simulink model "servo_motors_simulink"  (R2024b)
settings: Solver=VariableStepAuto  StartTime=0.0  StopTime=100  RelTol=1e-3
values from neighbouring files (symbols this model uses):
  Beq = Bm + Bt + B*r^2    (= 1)    [servo_motors_matlab.m]
  Jeq = Jm + Jt + M*r^2    (= 1)    [servo_motors_matlab.m]
  Kt = 1    [servo_motors_matlab.m]
libraries: slpidlib x4
settings Model: Creator=mstfy  LastModifiedBy=mstfy

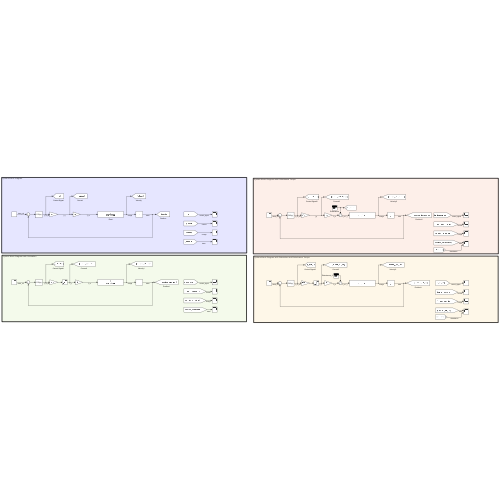
[thumbnail: Simulink's stored preview of the top-level diagram]
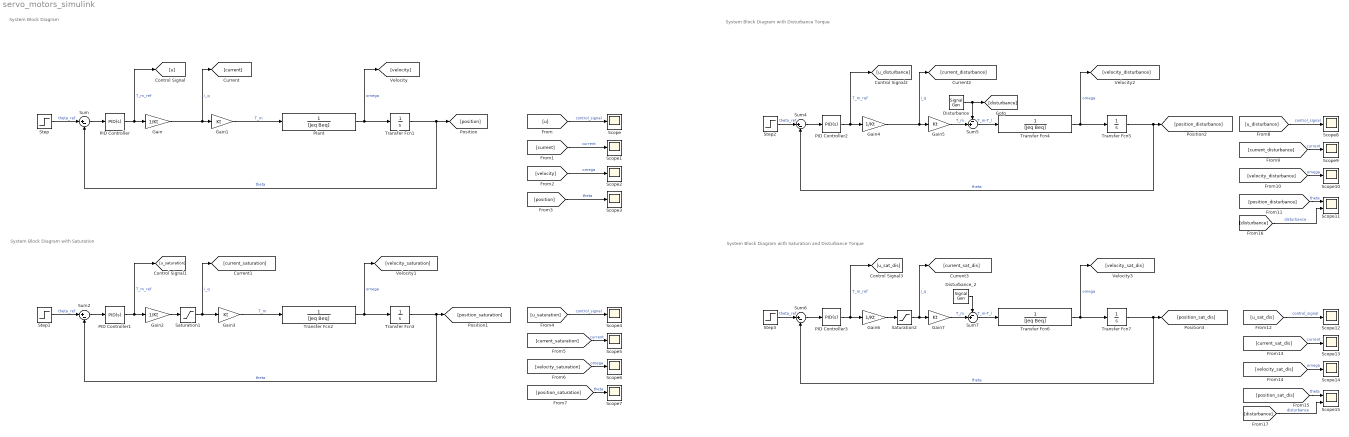
== system servo_motors_simulink ==
  note: System Block Diagram with Saturation
  note: System Block Diagram
  note: System Block Diagram with Disturbance Torque
  note: System Block Diagram with Saturation and Disturbance Torque
  Disturbance : SignalGenerator  WaveForm=square  Frequency=0.125  Units=rad/sec
  Disturbance_2 : SignalGenerator  WaveForm=square  Amplitude=0.5  Frequency=0.125  Units=rad/sec
  Gain{,2,4,6} (4 alike) : Gain  Gain=1/Kt
  Gain{1,3,5,7} (4 alike) : Gain  Gain=Kt
  PID Controller{,1..3} (4 alike) : slpidlib/PID Controller  Controller=PID  Form=Parallel  TimeDomain=Continuous-time  UseExternalTs=off  SampleTime=-1  IntegratorMethod=Forward Euler  FilterMethod=Forward Euler  ControllerParametersSource=internal  P=2.75  I=0.625  UseKiTs=off  D=2.5  UseExternalDerivativeSource=off  N=100  UseFilter=on  TunerSelectOption=Transfer Function Based (PID Tuner App)  InitialConditionSource=internal  InitialConditionForIntegrator=0  InitialConditionForFilter=0  DifferentiatorICPrevScaledInput=0  ExternalReset=none  TrackingMode=off  Kt=1  LimitOutput=off  SatLimitsSource=internal  UpperSaturationLimit=inf  LowerSaturationLimit=-inf  LinearizeAsGain=on  AntiWindupMode=none  Kb=1  LimitIntegrator=off  UpperIntegratorSaturationLimit=inf  LowerIntegratorSaturationLimit=-inf  POutMin=[]  POutMax=[]  IOutMin=[]  IOutMax=[]  DOutMin=[]  DOutMax=[]  NOutMin=[]  NOutMax=[]  SumOutMin=[]  SumOutMax=[]  SaturationOutMin=[]  SaturationOutMax=[]  PParamMin=[]  PParamMax=[]  IParamMin=[]  IParamMax=[]  DParamMin=[]  DParamMax=[]  NParamMin=[]  NParamMax=[]  KbParamMin=[]  KbParamMax=[]  KtParamMin=[]  KtParamMax=[]  KbOutMin=[]  KbOutMax=[]  KtOutMin=[]  KtOutMax=[]  IntegratorOutMin=[]  IntegratorOutMax=[]  FilterOutMin=[]  FilterOutMax=[]  SumI1OutMin=[]  SumI1OutMax=[]  SumI2OutMin=[]  SumI2OutMax=[]  SumI3OutMin=[]  SumI3OutMax=[]  SumI4OutMin=[]  SumI4OutMax=[]  SumDOutMin=[]  SumDOutMax=[]  DifferentiatorOutMin=[]  DifferentiatorOutMax=[]  FilterDiffOutCoefMin=[]  FilterDiffOutCoefMax=[]  ReciprocalOutMin=[]  ReciprocalOutMax=[]  SumDenOutMin=[]  SumDenOutMax=[]  SumNumOutMin=[]  SumNumOutMax=[]  DivideOutMin=[]  DivideOutMax=[]  UdiffTsProdOutMin=[]  UdiffTsProdOutMax=[]  NTsProdOutMin=[]  NTsProdOutMax=[]  UintegralTsProdOutMin=[]  UintegralTsProdOutMax=[]  UngainTsProdOutMin=[]  UngainTsProdOutMax=[]  ClampingZeroOutDataTypeStr=Inherit: Inherit via back propagation  ClampingZeroOutMin=[]  ClampingZeroOutMax=[]  FilterDenConstantOutDataTypeStr=Inherit: Inherit via back propagation  FilterDenConstantOutMin=[]  FilterDenConstantOutMax=[]  PCopyOutDataTypeStr=Inherit: Inherit via back propagation  PCopyOutMin=[]  PCopyOutMax=[]  NCopyOutDataTypeStr=Inherit: Inherit via back propagation  NCopyOutMin=[]  NCopyOutMax=[]  IntegratorContinuousStateAttributes=''  IntegratorStateMustResolveToSignalObject=off  IntegratorRTWStateStorageClass=Auto  FilterContinuousStateAttributes=''  FilterStateMustResolveToSignalObject=off  FilterRTWStateStorageClass=Auto  ParallelPVariant=InternalParameters  IdealPVariant=Disabled  IVariant=InternalParameters  DVariant=InternalParameters  IntegratorVariant=Continuous  SatVariant=Disabled  AWVariant=Passthrough  PCopyVariant=Disabled  TRVariant=Disabled  FdbkBlocksVariant=Forward  IdealPFdbkVariant=Disabled  SatFdbkVariant=Disabled  DerivativeFilterVariant=ContFilter  NVariant=InternalParameters  NCopyVariant=Disabled  FilterICVariant=InternalICsFilter  IntegratorICVariant=InternalICs  ExternalResetVariant=Disabled  TRSumVariant=Passthrough  SumFdbkVariant=Disabled  SumVariant=Sum_PID  TsampFilterVariant=InternalTs  TsampNgainVariant=Passthrough  TsampIntegralVariant=Disabled_SignalSpec  ExternalSaturationOutDataTypeStr=Inherit: Same as second input  DerivativeSourceVariant=ErrorSignal  PreIntVariant=InternalPreInt
  Plant : TransferFcn  Denominator=[Jeq Beq]
  Saturation1 : Saturate  UpperLimit=20  LowerLimit=-20
  Saturation2 : Saturate  UpperLimit=20  LowerLimit=-20
  Scope{,1..10,12..14} (14 alike) : Scope
  Scope11 : Scope  NumInputPorts=2
  Scope15 : Scope  NumInputPorts=2
  Step{,1..3} (4 alike) : Step  Time=0  SampleTime=0
  Sum{,2,4,6} (4 alike) : Sum  Inputs=|+-
  Sum5 : Sum  Inputs=-+|
  Sum7 : Sum  Inputs=-+|
  Transfer Fcn{1,3,5,7} (4 alike) : TransferFcn  Denominator=[1 0]
  Transfer Fcn2 : TransferFcn  Denominator=[Jeq Beq]
  Transfer Fcn4 : TransferFcn  Denominator=[Jeq Beq]
  Transfer Fcn6 : TransferFcn  Denominator=[Jeq Beq]
  wires:
  Step/1 -> Sum/1  "theta_ref"
  Sum/1 -> PID Controller/1
  PID Controller/1 -> [u], Gain/1  "T_m_ref"
  Gain1/1 -> Plant/1  "T_m"
  Plant/1 -> [velocity], Transfer Fcn1/1  "omega"
  Transfer Fcn1/1 -> [position], Sum/2  "theta"
  Gain/1 -> [current], Gain1/1  "i_q"
  [velocity] -> Scope2/1  "omega"
  [position] -> Scope3/1  "theta"
  [current] -> Scope1/1  "current"
  [u] -> Scope/1  "control_signal"
  [position_saturation] -> Scope7/1  "theta"
  Transfer Fcn3/1 -> Sum2/2, [position_saturation]  "theta"
  Gain3/1 -> Transfer Fcn2/1  "T_m"
  [current_saturation] -> Scope5/1  "current"
  Sum2/1 -> PID Controller1/1
  [velocity_saturation] -> Scope6/1  "omega"
  PID Controller1/1 -> [u_saturation], Gain2/1  "T_m_ref"
  Gain2/1 -> Saturation1/1
  Step1/1 -> Sum2/1  "theta_ref"
  Saturation1/1 -> [current_saturation], Gain3/1  "i_q"
  [u_saturation] -> Scope4/1  "control_signal"
  Transfer Fcn2/1 -> [velocity_saturation], Transfer Fcn3/1  "omega"
  PID Controller3/1 -> [u_sat_dis], Gain6/1  "T_m_ref"
  Step3/1 -> Sum6/1  "theta_ref"
  [u_sat_dis] -> Scope12/1  "control_signal"
  Saturation2/1 -> [current_sat_dis], Gain7/1  "i_q"
  Gain5/1 -> Sum5/2  "T_m"
  Gain6/1 -> Saturation2/1
  Transfer Fcn6/1 -> [velocity_sat_dis], Transfer Fcn7/1  "omega"
  Transfer Fcn7/1 -> Sum6/2, [position_sat_dis]  "theta"
  Sum6/1 -> PID Controller3/1
  Gain7/1 -> Sum7/2  "T_m"
  [velocity_sat_dis] -> Scope14/1  "omega"
  [position_disturbance] -> Scope11/1  "theta"
  Sum7/1 -> Transfer Fcn6/1  "T_m-T_l"
  Transfer Fcn5/1 -> Sum4/2, [position_disturbance]  "theta"
  Gain4/1 -> [current_disturbance], Gain5/1  "i_q"
  Sum5/1 -> Transfer Fcn4/1  "T_m-T_l"
  [current_disturbance] -> Scope9/1  "current"
  Sum4/1 -> PID Controller2/1
  [velocity_disturbance] -> Scope10/1  "omega"
  PID Controller2/1 -> [u_disturbance], Gain4/1  "T_m_ref"
  Step2/1 -> Sum4/1  "theta_ref"
  [current_sat_dis] -> Scope13/1  "current"
  [position_sat_dis] -> Scope15/1  "theta"
  [u_disturbance] -> Scope8/1  "control_signal"
  Transfer Fcn4/1 -> [velocity_disturbance], Transfer Fcn5/1  "omega"
  Disturbance/1 -> [disturbance], Sum5/1
  Disturbance_2/1 -> Sum7/1
  [disturbance] -> Scope11/2  "disturbance"
  [disturbance] -> Scope15/2  "disturbance"
